simulink model "Ro_Po_Calculation"  (R2024a)
settings: Solver=VariableStepAuto  StartTime=0.0  StopTime=10.0  RelTol=1e-3
settings Model: Creator=ACER  LastModifiedBy=ACER

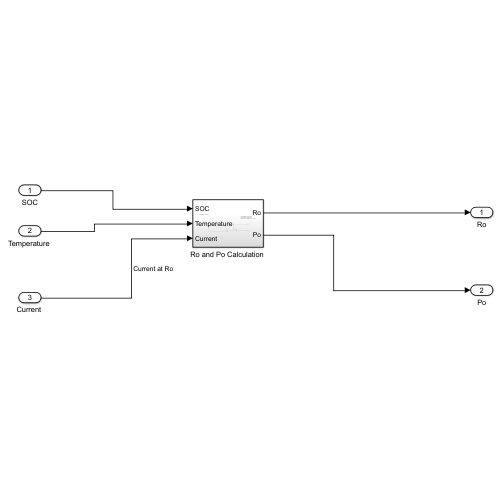
[thumbnail: Simulink's stored preview of the top-level diagram]
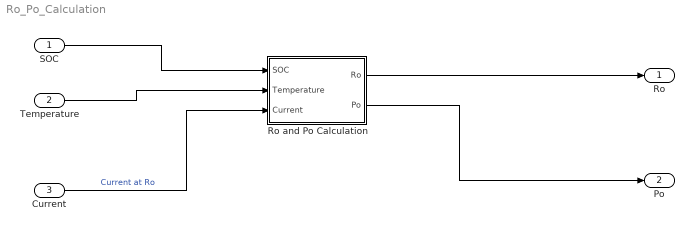
== system Ro_Po_Calculation ==
  SOC : Inport
  "Temperature " : Inport  Port=2
  "Current " : Inport  Port=3
  "Ro and Po Calculation " : Subsystem
  Ro : Outport
  Po : Outport  Port=2
  wires:
  SOC/1 -> "Ro and Po Calculation "/1(SOC)
  "Temperature "/1 -> "Ro and Po Calculation "/2("Temperature ")
  "Current "/1 -> "Ro and Po Calculation "/3("Current ")  "Current at Ro"
  "Ro and Po Calculation "/1(Ro) -> Ro/1
  "Ro and Po Calculation "/2(Po) -> Po/1

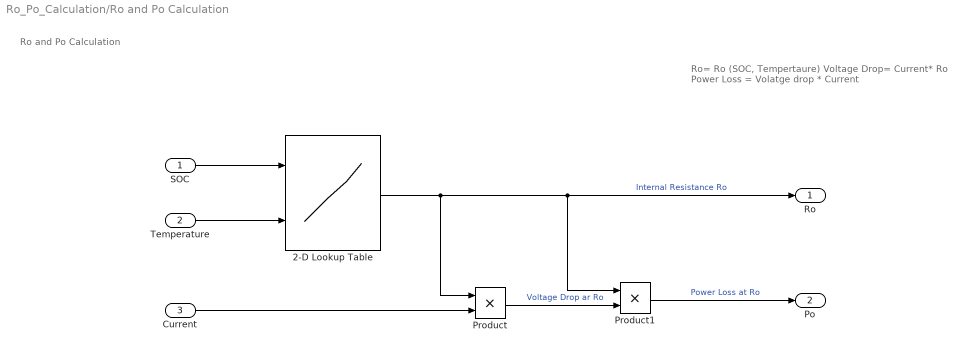
== system Ro_Po_Calculation/Ro and Po Calculation  ==
  note: Ro= Ro (SOC, Tempertaure)
      | Voltage Drop= Current* Ro
      | Power Loss = Volatge drop * Current
  note: Ro and Po Calculation
  SOC : Inport
  "Temperature " : Inport  Port=2
  "Current " : Inport  Port=3
  2-D Lookup Table : Lookup_n-D  BreakpointsForDimension1=[1:3]  BreakpointsForDimension2=[1:3]  InternalRulePriority=Speed  RndMeth=Simplest
      settings: InputPortMap=u0,u1
  Product : Product
  Product1 : Product
  Ro : Outport
  Po : Outport  Port=2
  wires:
  Product1/1 -> Po/1  "Power Loss at Ro"
  2-D Lookup Table/1 -> Ro/1, Product1/1, Product/1  "Internal Resistance Ro"
  "Temperature "/1 -> 2-D Lookup Table/2
  "Current "/1 -> Product/2
  Product/1 -> Product1/2  "Voltage Drop ar Ro"
  SOC/1 -> 2-D Lookup Table/1
